simulink subsystem "DCDCConverterSSC"  (R2022b)
settings: Solver=VariableStepAuto  StartTime=0.0  StopTime=10.0  RelTol=1e-3
undefined symbols (not defined in the file): PlntBattNumCellSer, PlntBattOpenCirctVolt, PlntBattSocInit, PlntBattVoltSocBpt
libraries: fl_lib x3, ee_lib x1
settings Model: Creator=The MathWorks, Inc.  LastModifiedBy=The MathWorks, Inc.

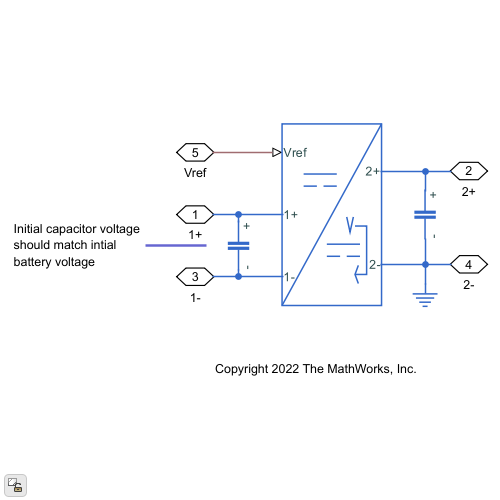
[thumbnail: Simulink's stored preview of the top-level diagram]
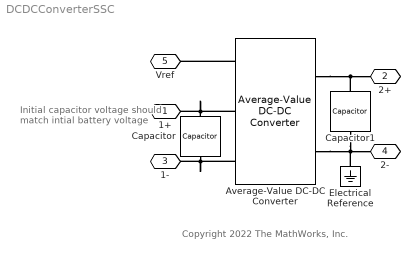
== system DCDCConverterSSC ==
  note: Initial capacitor voltage
      | should match intial
      | battery voltage
  note: Copyright 2022 The MathWorks, Inc.
  Average-Value DC-DC Converter : ee_lib/Semiconductors & Converters/Converters/Average-Value DC-DC Converter  control_option=ee.enum.converters.controlinput.voltage  converter_type=ee.enum.converters.dcdctype.buck  efficiency_option=ee.enum.converters.efficiency.constant  efficiency_fixed=PlntDCDCEff  i_vec=[0, 2, 5] A  efficiency_vec=[90, 95, 98]
      settings: InternalSimscapePortConfiguration="{\"Bottom\":[],\"Left\":[{\"id\":\"Vref\",\"label\":\"Vref\",\"type\":\"input\"},{\"id\":\"p1\",\"label\":\"1+\",\"type\":\"foundation.electrical.electrical\"},{\"id\":\"n1\",\"label\":\"1-\",\"type\":\"foundation.electrical.electrical\"}],\"Right\":[{\"id\":\"p2\",\"label\":\"2+\",\"type\":\"foundation.electrical.electrical\"},{\"id\":\"n2\",\"label\":\"2-\",\"type\":\"foundation.electrical.electrical\"}],\"Top\":[]}"
  Capacitor : fl_lib/Electrical/Electrical Elements/Capacitor  c=PlntDCDCFltrCap uF  r=PlntDCDCFltrRes Ohm  g=0 1/Ohm  i_specify=off  i_priority=None  i=0 A  i_nominal_specify=off  i_nominal_unit=A  i_nominal_value=1  v_specify=off  v_priority=None  v=0 V  v_nominal_specify=off  v_nominal_unit=V  v_nominal_value=1  vc_specify=on  vc_priority=High  vc=interp1(PlntBattVoltSocBpt, PlntBattOpenCirctVolt, PlntBattSocInit)*PlntBattNumCellSer V  vc_nominal_specify=off  vc_nominal_unit=V  vc_nominal_value=1
  Capacitor1 : fl_lib/Electrical/Electrical Elements/Capacitor  c=PlntDCDCFltrCap uF  r=PlntDCDCFltrRes Ohm  g=0 1/Ohm  i_specify=off  i_priority=None  i=0 A  i_nominal_specify=off  i_nominal_unit=A  i_nominal_value=1  v_specify=off  v_priority=None  v=0 V  v_nominal_specify=off  v_nominal_unit=V  v_nominal_value=1  vc_specify=on  vc_priority=High  vc=PlntDCDCVoltInit V  vc_nominal_specify=off  vc_nominal_unit=V  vc_nominal_value=1
  Electrical Reference : fl_lib/Electrical/Electrical Elements/Electrical Reference
  1+ : PMIOPort  Side=Left
  2+ : PMIOPort  Port=2  Side=Right
  1- : PMIOPort  Port=3  Side=Left
  2- : PMIOPort  Port=4  Side=Right
  Vref : PMIOPort  Port=5  Side=Left
  connections:
  Electrical Reference/LConn1 -- Average-Value DC-DC Converter/RConn2 -- Capacitor1/RConn1 -- 2-/RConn1
  Average-Value DC-DC Converter/LConn1 -- Vref/RConn1
  Average-Value DC-DC Converter/LConn3 -- Capacitor/RConn1 -- 1-/RConn1
  Average-Value DC-DC Converter/RConn1 -- Capacitor1/LConn1 -- 2+/RConn1
  Capacitor/LConn1 -- Average-Value DC-DC Converter/LConn2 -- 1+/RConn1
